simulink model "kalman_current_and_wave_disturbances"  (R2017a)
settings: Solver=ode45  StartTime=0.0  StopTime=1000  RelTol=1e-3  EnableMultiTasking=on
values from neighbouring files (symbols this model uses):
  K_pd = sqrt(w_c^2 + T_f^2 * w_c^4)/K    [kalman_current_and_wave_disturbances_init.m]    (also in kalman_current_and_wave_noise_init.m)
  T_d = T    (= 72.442)    [kalman_current_and_wave_disturbances_init.m]    (also in kalman_current_and_wave_noise_init.m)
  T_f = 1/(w_c * tan(-130*(pi/180)))    [kalman_current_and_wave_disturbances_init.m]    (also in kalman_current_and_wave_noise_init.m)
undefined symbols (not defined in the file): m
libraries: simulink x2
settings Model: Creator=markh  LastModifiedBy=simenrau
settings DataIOCC: LimitDataPoints=on  SaveFormat=Array  SignalLoggingSaveFormat=ModelDataLogs  SignalLoggingName=sigsOut
settings OptimizationCC: InitFltsAndDblsToZero=on  LifeSpan=inf
settings DebuggingCC: SaveWithParameterizedLinksMsg=none  UnderspecifiedInitializationDetection=Classic  MergeDetectMultiDrivingBlocksExec=none  SignalResolutionControl=TryResolveAllWithWarning  MultiTaskDSMMsg=warning  MultiTaskCondExecSysMsg=none  FcnCallInpInsideContextMsg=warning  StateNameClashWarn=warning  SFUnexpectedBacktrackingDiag=warning  SFNoUnconditionalDefaultTransitionDiag=warning  SFExecutionAtInitializationDiag=none
settings HardwareCC: ProdBitPerPointer=32  ProdBitPerSizeT=32  ProdBitPerPtrDiffT=32  ProdLargestAtomicFloat=None  ProdIntDivRoundTo=Undefined  ProdEndianess=Unspecified  ProdWordSize=32  ProdHWDeviceType=32-bit Generic  TargetUnknown=on
settings ModelReferenceCC: PropagateSignalLabelsOutOfModel=off
settings GRTTargetCC: TargetFcnLib=ansi_tfl_tmw.mat  TargetLangStandard=C89/C90 (ANSI)  GeneratePreprocessorConditionals=Disable all  CombineOutputUpdateFcns=off  GRTInterface=on
settings ConfigComp: CovMetricSettings=dw  CovHtmlReporting=on  CovSaveCumulativeToWorkspaceVar=on  CovSaveSingleToWorkspaceVar=on  CovExternalEMLEnable=off

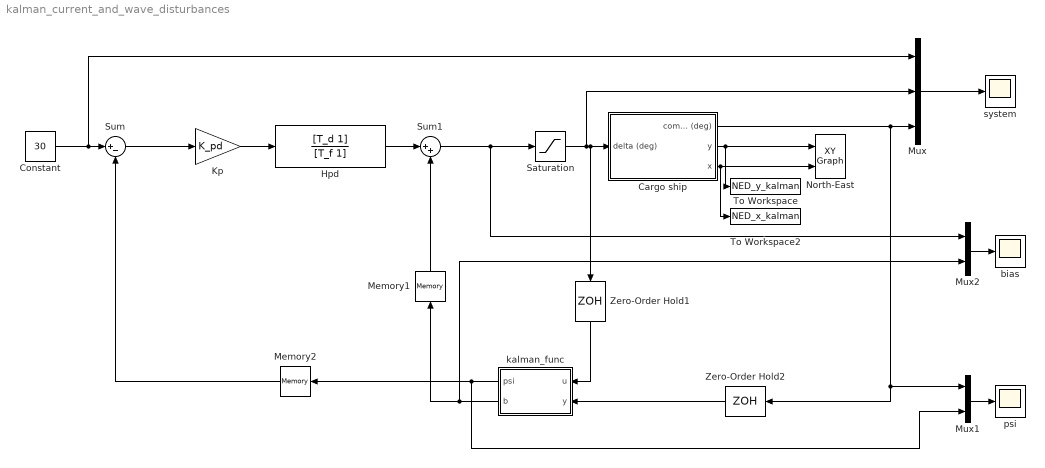
== system kalman_current_and_wave_disturbances ==
  Cargo ship : Subsystem  mask(Simple shipmodel for a cargo ship){noise=off, current=off, logic=off}
      mask prompts: noise "measurement noise"; logic "waves"
      mask help:
      | Measurement noise:
      | 	checked = noise on
      | 	unchecked = noise off
      |
      | Current:
      | 	checked = current on
      | 	unchecked = current off
      |
      | Waves:
      | 	checked = waves on
      | 	unchecked = waves off
      |
      | Author: Jørgen Spjøtvold, 9/10-2003
      | TTK 4115 Linear system theory.
      | Modified by Jostein Bakkeheim 26/10-2006
  Constant : Constant  Value=30
  Hpd : TransferFcn  Numerator=[T_d 1]  Denominator=[T_f 1]
  Kp : Gain  Gain=K_pd
  Memory1 : Memory
  Memory2 : Memory
  Mux : Mux  Inputs=3
  Mux1 : Mux  Inputs=2
  Mux2 : Mux  Inputs=2
  North-East : simulink/Sinks/XY Graph  xmin=-5000  xmax=5000  ymin=-5000  ymax=5000  st=-1
  Saturation : Saturate  UpperLimit=35  LowerLimit=-35
  Sum : Sum  Inputs=|+-
  Sum1 : Sum  Inputs=|++
  To Workspace : ToWorkspace  VariableName=NED_y_kalman  SampleTime=-1
  To Workspace2 : ToWorkspace  VariableName=NED_x_kalman  SampleTime=-1
  Zero-Order Hold1 : ZeroOrderHold  SampleTime=0.1
  Zero-Order Hold2 : ZeroOrderHold  SampleTime=0.1
  bias : Scope
  "kalman_func " : MATLAB Function  TreatAsAtomicUnit=on  mask{m=m}
      mask prompts: m "struct m"
  psi : Scope
  system : Scope
  wires:
  Cargo ship/3(x) -> North-East/2, To Workspace2/1
  Cargo ship/2(y) -> North-East/1, To Workspace/1
  Kp/1 -> Hpd/1
  Mux/1 -> system/1
  Sum/1 -> Kp/1
  Saturation/1 -> Zero-Order Hold1/1, Cargo ship/1(delta (deg)), Mux/2
  Constant/1 -> Mux/1, Sum/1
  Hpd/1 -> Sum1/1
  Sum1/1 -> Saturation/1, Mux2/1
  Zero-Order Hold1/1 -> "kalman_func "/1(u)
  Zero-Order Hold2/1 -> "kalman_func "/2(y)
  Cargo ship/1(compass (deg)) -> Zero-Order Hold2/1, Mux1/1, Mux/3
  Memory1/1 -> Sum1/2
  "kalman_func "/2(b) -> Memory1/1, Mux2/2
  "kalman_func "/1(psi) -> Memory2/1, Mux1/2
  Memory2/1 -> Sum/2
  Mux1/1 -> psi/1
  Mux2/1 -> bias/1

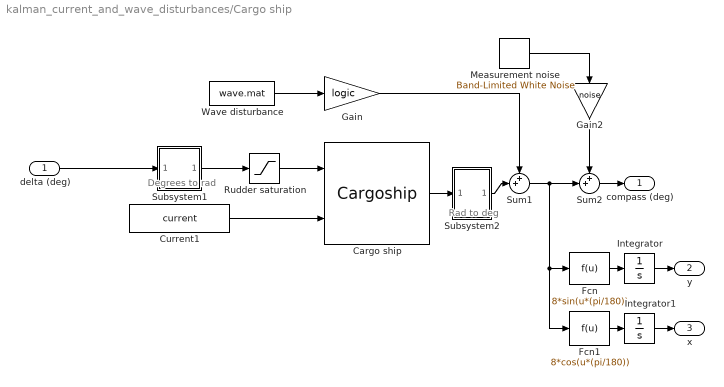
== system kalman_current_and_wave_disturbances/Cargo ship ==
  note: Degrees to rad
  note: Rad to deg
  delta (deg) : Inport
  Cargo ship : S-Function  FunctionName=Cargoship  SFunctionDeploymentMode=off  EnableBusSupport=off  mask(Cargo ship){}
      mask help:
      | S-function which simulates a cargo ship.
      |
      | Author: Jørgen Spjøtvold
      | 20.10-2003
      | Modified by Jostein Bakkeheim 27.10.2006
  Current1 : Constant  Value=current
  Fcn : Fcn  Expr=8*sin(u*(pi/180))
  Fcn1 : Fcn  Expr=8*cos(u*(pi/180))
  Gain : Gain  Gain=logic  SaturateOnIntegerOverflow=on  OutDataTypeStr=Inherit: Same as input  ParamDataTypeStr=Inherit: Same as input
  Gain2 : Gain  Gain=noise  SaturateOnIntegerOverflow=on  OutDataTypeStr=Inherit: Same as input  ParamDataTypeStr=Inherit: Same as input
  Integrator : Integrator
  Integrator1 : Integrator
  Measurement noise : simulink/Sources/Band-Limited White Noise  Cov=[0.001]  Ts=.5  seed=[23341]
  Rudder saturation : Saturate  UpperLimit=45*(pi/180)  LowerLimit=-45*(pi/180)
  Subsystem1 : Subsystem  mask(degrees to radians){}
      mask help: Converts degrees to radians
      mask Display: fprintf('D2R');
  Subsystem2 : Subsystem  mask(radians to degrees){}
      mask help: Converts radians to degrees
      mask Display: fprintf('R2D');
  Sum1 : Sum  Inputs=++|  SaturateOnIntegerOverflow=on
  Sum2 : Sum  Inputs=++|  SaturateOnIntegerOverflow=on
  Wave disturbance : FromFile  FileName=wave.mat  SampleTime=0
  compass (deg) : Outport
  y : Outport  Port=2
  x : Outport  Port=3
  wires:
  delta (deg)/1 -> Subsystem1/1(In1)
  Fcn/1 -> Integrator/1
  Integrator/1 -> y/1
  Fcn1/1 -> Integrator1/1
  Integrator1/1 -> x/1
  Wave disturbance/1 -> Gain/1
  Subsystem2/1(Out1) -> Sum1/2
  Gain/1 -> Sum1/1
  Sum1/1 -> Fcn/1, Fcn1/1, Sum2/2
  Cargo ship/1 -> Subsystem2/1(In1)
  Subsystem1/1(Out1) -> Rudder saturation/1
  Rudder saturation/1 -> Cargo ship/1
  Sum2/1 -> compass (deg)/1
  Measurement noise/1 -> Gain2/1
  Gain2/1 -> Sum2/1
  Current1/1 -> Cargo ship/2

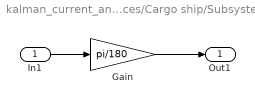
== system kalman_current_and_wave_disturbances/Cargo ship/Subsystem1 ==
  In1 : Inport
  Gain : Gain  Gain=pi/180  SaturateOnIntegerOverflow=on  OutDataTypeStr=Inherit: Same as input  ParamDataTypeStr=Inherit: Same as input
  Out1 : Outport
  wires:
  Gain/1 -> Out1/1
  In1/1 -> Gain/1

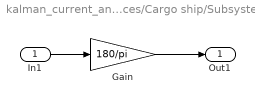
== system kalman_current_and_wave_disturbances/Cargo ship/Subsystem2 ==
  In1 : Inport
  Gain : Gain  Gain=180/pi  SaturateOnIntegerOverflow=on  OutDataTypeStr=Inherit: Same as input  ParamDataTypeStr=Inherit: Same as input
  Out1 : Outport
  wires:
  Gain/1 -> Out1/1
  In1/1 -> Gain/1

== matlab function kalman_current_and_wave_disturbances/kalman_func  ==
  data: u input; psi output; y input; b output; m parameter
function [psi, b] = kalman_func(u, y, m)

persistent init_flag A B C D E Q R P_minus x_minus I

if isempty(init_flag)
init_flag=1;

A = m.A;
B = m.B;
C = m.C;
D = m.D; 
E = m.E;
Q = m.Q;
R = m.R;
P_minus = m.P_0;
x_minus = m.x_0;
I = m.I;
end

L = P_minus*C'*(C*P_minus*C' + R)^-1;

P = (I - L*C)*P_minus*(I - L*C)' + L*R*L';

x = x_minus + L*(y - C*x_minus);

x_minus = A*x + B*u;
P_minus = A*P*A' + E*Q*E';

psi = x(3); 
b = x(5);

end
